simulink model "compare1"  (R2024b)
settings: Solver=VariableStepAuto  StartTime=0.0  StopTime=10.0  RelTol=1e-3
libraries: simulink x15
settings Model: Creator=Ahmad  LastModifiedBy=Ahmad

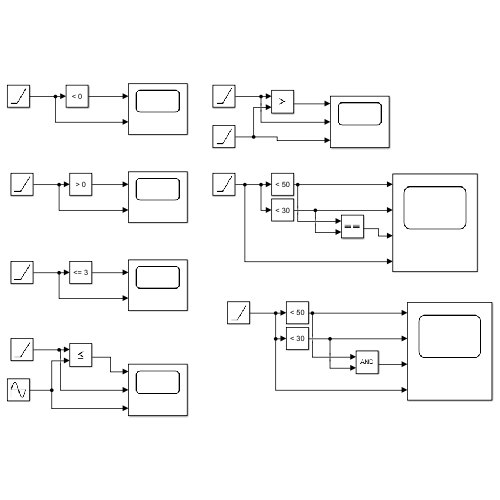
[thumbnail: Simulink's stored preview of the top-level diagram]
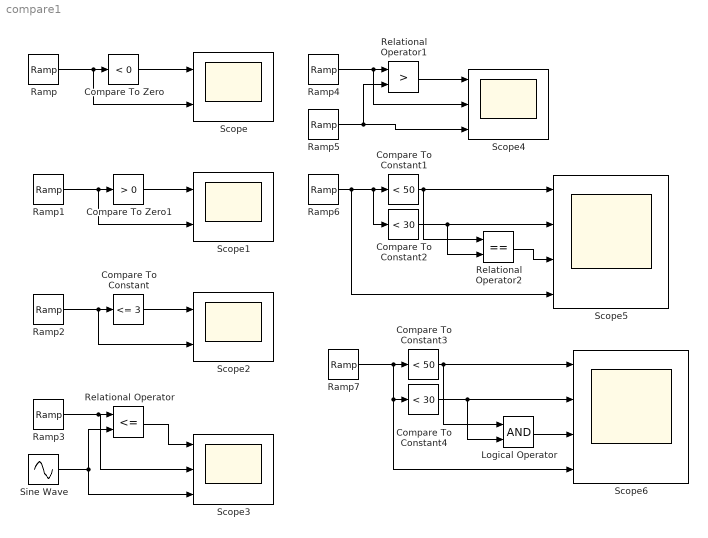
== system compare1 ==
  Compare To Constant : simulink/Logic and Bit Operations/Compare To Constant  relop=<=  const=3  OutDataTypeStr=boolean
  Compare To Constant1 : simulink/Logic and Bit Operations/Compare To Constant  relop=<  const=50  OutDataTypeStr=boolean
  Compare To Constant2 : simulink/Logic and Bit Operations/Compare To Constant  relop=<  const=30  OutDataTypeStr=boolean
  Compare To Constant3 : simulink/Logic and Bit Operations/Compare To Constant  relop=<  const=50  OutDataTypeStr=boolean
  Compare To Constant4 : simulink/Logic and Bit Operations/Compare To Constant  relop=<  const=30  OutDataTypeStr=boolean
  Compare To Zero : simulink/Logic and Bit Operations/Compare To Zero  relop=<  OutDataTypeStr=boolean
  Compare To Zero1 : simulink/Logic and Bit Operations/Compare To Zero  relop=>  OutDataTypeStr=boolean
  Logical Operator : Logic  AllPortsSameDT=off  OutDataTypeStr=boolean
  Ramp : simulink/Sources/Ramp  slope=-1  start=3  InitialOutput=0
  Ramp{1..4} (4 alike) : simulink/Sources/Ramp  slope=1  start=3  InitialOutput=0
  Ramp5 : simulink/Sources/Ramp  slope=1  start=5  InitialOutput=0
  Ramp6 : simulink/Sources/Ramp  slope=30  start=3  InitialOutput=0
  Ramp7 : simulink/Sources/Ramp  slope=30  start=3  InitialOutput=0
  Relational Operator : RelationalOperator  Operator=<=  OutDataTypeStr=boolean  RndMeth=Simplest  InputSameDT=off
  Relational Operator1 : RelationalOperator  Operator=>  OutDataTypeStr=boolean  RndMeth=Simplest  InputSameDT=off
  Relational Operator2 : RelationalOperator  Operator===  OutDataTypeStr=boolean  RndMeth=Simplest  InputSameDT=off
  Scope : Scope  NumInputPorts=2
  Scope1 : Scope  NumInputPorts=2
  Scope2 : Scope  NumInputPorts=2
  Scope3 : Scope  NumInputPorts=3
  Scope4 : Scope  NumInputPorts=3
  Scope5 : Scope  NumInputPorts=4
  Scope6 : Scope  NumInputPorts=4
  Sine Wave : Sin  SampleTime=0
  wires:
  Ramp/1 -> Scope/2, Compare To Zero/1
  Compare To Zero/1 -> Scope/1
  Compare To Zero1/1 -> Scope1/1
  Ramp1/1 -> Scope1/2, Compare To Zero1/1
  Ramp2/1 -> Scope2/2, Compare To Constant/1
  Compare To Constant/1 -> Scope2/1
  Ramp3/1 -> Scope3/2, Relational Operator/1
  Sine Wave/1 -> Scope3/3, Relational Operator/2
  Relational Operator/1 -> Scope3/1
  Ramp5/1 -> Scope4/3, Relational Operator1/2
  Ramp4/1 -> Scope4/2, Relational Operator1/1
  Relational Operator1/1 -> Scope4/1
  Compare To Constant1/1 -> Relational Operator2/1, Scope5/1
  Compare To Constant2/1 -> Relational Operator2/2, Scope5/2
  Relational Operator2/1 -> Scope5/3
  Ramp6/1 -> Scope5/4, Compare To Constant2/1, Compare To Constant1/1
  Ramp7/1 -> Compare To Constant4/1, Scope6/4, Compare To Constant3/1
  Compare To Constant4/1 -> Logical Operator/2, Scope6/2
  Compare To Constant3/1 -> Logical Operator/1, Scope6/1
  Logical Operator/1 -> Scope6/3
